simulink model "ExampleAlphaMesh"  (R2024a)
settings: Solver=FixedStepAuto  StartTime=0.0  StopTime=inf  FixedStep=0.02  RelTol=1e-3  EnableMultiTasking=on
undefined symbols (not defined in the file): atmosphericScattering, basicProperties, castShadow, emissionColorMultiplier, meshID, position, quaternion, scale, visible
libraries: PRISMA x14, GenericTarget x1
settings Model: Creator=damerius  LastModifiedBy=Scythe
settings SolverCC: ConcurrentTasks=on  AlgebraicLoopSolver=TrustRegion  PositivePriorityOrder=on
settings DataIOCC: SaveOutput=off  SignalLogging=off  DSMLogging=off  SaveTime=off  ReturnWorkspaceOutputs=off
settings OptimizationCC: DefaultParameterBehavior=Inlined  ReuseModelBlockBuffer=off  ZeroExternalMemoryAtStartup=off  ZeroInternalMemoryAtStartup=off  SimCompilerOptimization=on
settings DebuggingCC: UnconnectedInputMsg=warning  UnconnectedOutputMsg=warning  UnconnectedLineMsg=warning
settings HardwareCC: ProdBitPerLong=64  ProdHWDeviceType=Intel->x86-64 (Linux 64)
settings ModelReferenceCC: EnableRefExpFcnMdlSchedulingChecks=on
settings SFSimCC: SimParseCustomCode=off  SimGenImportedTypeDefs=on  SimTargetLang=C++
settings RTWCC: GenCodeOnly=on  PackageGeneratedCodeAndArtifacts=on  PackageName=PackNGo  RTWVerbose=off  BuildConfiguration=Faster Runs  TargetLang=C++  GPUComputeCapability=3.5  DLArmComputeVersion=19.05
settings CodeAppCC: ForceParamTrailComments=on  MaxIdLength=95  MATLABSourceComments=on  UseSimReservedNames=on
settings GRTTargetCC: TargetLangStandard=C++11 (ISO)  GenerateFullHeader=off  MatFileLogging=off  CodeInterfacePackaging=C++ class

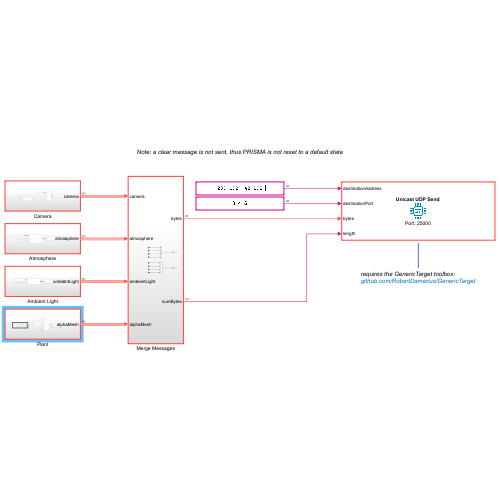
[thumbnail: Simulink's stored preview of the top-level diagram]
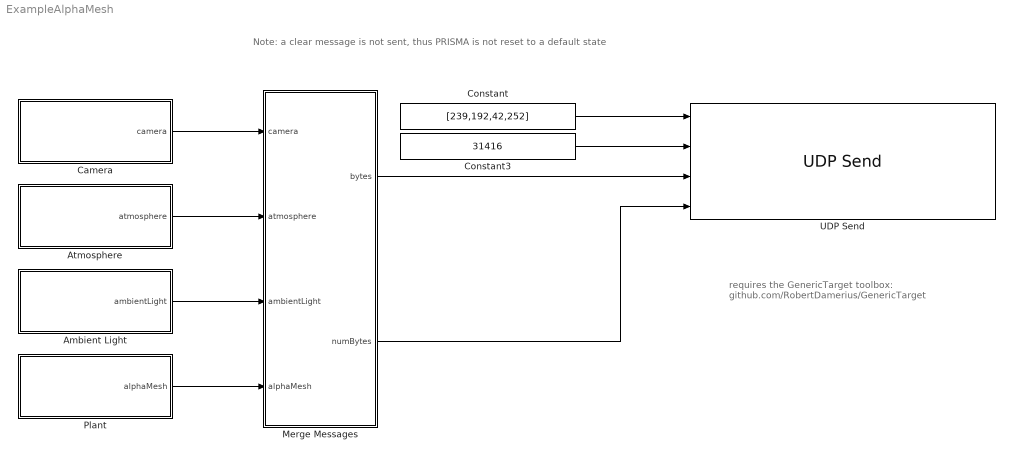
== system ExampleAlphaMesh ==
  note: Note: a clear message is not sent, thus PRISMA is not reset to a default state
  note: requires the GenericTarget toolbox:
      | github.com/RobertDamerius/GenericTarget
  Ambient Light : Subsystem
  Atmosphere : Subsystem
  Camera : Subsystem
  Constant : Constant  Value=[239,192,42,252]  OutDataTypeStr=uint8
  Constant3 : Constant  Value=31416  OutDataTypeStr=uint16
  Merge Messages : Subsystem
  Plant : Subsystem
  UDP Send : GenericTarget/Interface/UDP Send  showDetails=off  interfacePort=25000  interfaceIP=[0,0,0,0]  deviceName=''  prioritySocket=6  allowBroadcast=off  SampleTime=-1
      settings: SourceProductName=Generic Target
  wires:
  Constant3/1 -> UDP Send/2
  Camera/1(camera) -> Merge Messages/1(camera)
  Plant/1(alphaMesh) -> Merge Messages/4(alphaMesh)
  Merge Messages/1(bytes) -> UDP Send/3
  Merge Messages/2(numBytes) -> UDP Send/4
  Ambient Light/1(ambientLight) -> Merge Messages/3(ambientLight)
  Constant/1 -> UDP Send/1
  Atmosphere/1(atmosphere) -> Merge Messages/2(atmosphere)

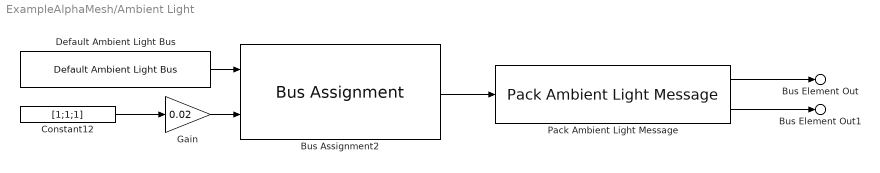
== system ExampleAlphaMesh/Ambient Light ==
  Bus Assignment2 : BusAssignment  AssignedSignals=color
  Constant12 : Constant  Value=[1;1;1]
  Default Ambient Light Bus : PRISMA/Default Ambient Light Bus
      settings: SourceProductName=PRISMA
  Gain : Gain  Gain=0.02
  Pack Ambient Light Message : PRISMA/Pack Ambient Light Message
      settings: SourceProductName=PRISMA
  Bus Element Out : Outport  PortName=ambientLight  Element=bytes
  Bus Element Out1 : Outport  PortName=ambientLight  Element=numBytes
  wires:
  Pack Ambient Light Message/2 -> Bus Element Out1/1
  Pack Ambient Light Message/1 -> Bus Element Out/1
  Gain/1 -> Bus Assignment2/2
  Constant12/1 -> Gain/1
  Default Ambient Light Bus/1 -> Bus Assignment2/1
  Bus Assignment2/1 -> Pack Ambient Light Message/1

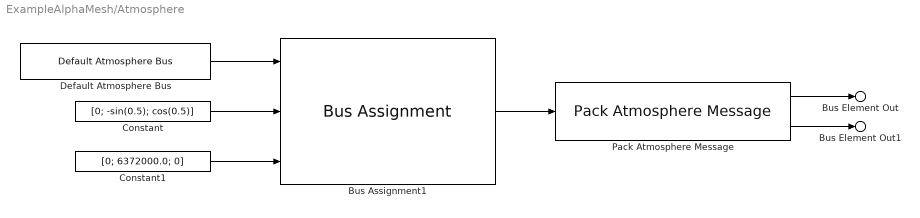
== system ExampleAlphaMesh/Atmosphere ==
  Bus Assignment1 : BusAssignment  AssignedSignals=basicProperties.sunLightDirection,atmosphericScattering.eyePosition
  Constant : Constant  Value=[0; -sin(0.5); cos(0.5)]
  Constant1 : Constant  Value=[0; 6372000.0; 0]
  Default Atmosphere Bus : PRISMA/Default Atmosphere Bus
      settings: SourceProductName=PRISMA
  Pack Atmosphere Message : PRISMA/Pack Atmosphere Message
      settings: SourceProductName=PRISMA
  Bus Element Out : Outport  PortName=atmosphere  Element=bytes
  Bus Element Out1 : Outport  PortName=atmosphere  Element=numBytes
  wires:
  Bus Assignment1/1 -> Pack Atmosphere Message/1
  Default Atmosphere Bus/1 -> Bus Assignment1/1
  Pack Atmosphere Message/1 -> Bus Element Out/1
  Pack Atmosphere Message/2 -> Bus Element Out1/1
  Constant/1 -> Bus Assignment1/2
  Constant1/1 -> Bus Assignment1/3

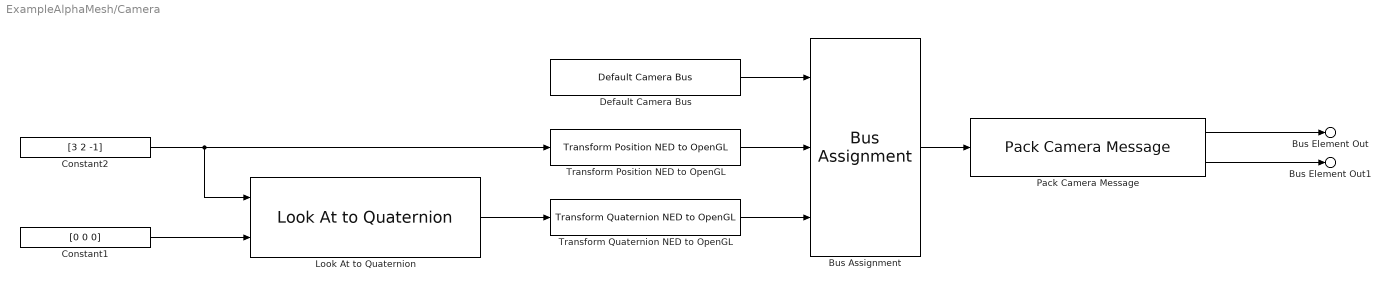
== system ExampleAlphaMesh/Camera ==
  Bus Assignment : BusAssignment  AssignedSignals=position,quaternion
  Constant1 : Constant  Value=[0 0 0]
  Constant2 : Constant  Value=[3 2 -1]
  Default Camera Bus : PRISMA/Default Camera Bus
      settings: SourceProductName=PRISMA
  Look At to Quaternion : PRISMA/Transformation/Look At to Quaternion
      settings: SourceProductName=PRISMA
  Pack Camera Message : PRISMA/Pack Camera Message
      settings: SourceProductName=PRISMA
  Transform Position NED to OpenGL : PRISMA/Transformation/Transform Position NED to OpenGL
      settings: SourceProductName=PRISMA
  Transform Quaternion NED to OpenGL : PRISMA/Transformation/Transform Quaternion NED to OpenGL
      settings: SourceProductName=PRISMA
  Bus Element Out : Outport  PortName=camera  Element=bytes
  Bus Element Out1 : Outport  PortName=camera  Element=numBytes
  wires:
  Default Camera Bus/1 -> Bus Assignment/1
  Bus Assignment/1 -> Pack Camera Message/1
  Transform Position NED to OpenGL/1 -> Bus Assignment/2
  Transform Quaternion NED to OpenGL/1 -> Bus Assignment/3
  Look At to Quaternion/1 -> Transform Quaternion NED to OpenGL/1
  Constant1/1 -> Look At to Quaternion/2
  Pack Camera Message/1 -> Bus Element Out/1
  Pack Camera Message/2 -> Bus Element Out1/1
  Constant2/1 -> Look At to Quaternion/1, Transform Position NED to OpenGL/1

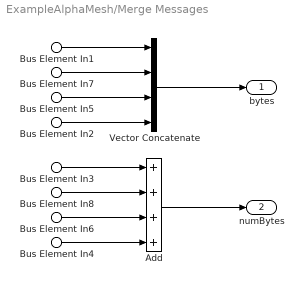
== system ExampleAlphaMesh/Merge Messages ==
  Bus Element In1 : Inport  PortName=camera  Element=bytes
  Bus Element In3 : Inport  PortName=camera  Element=numBytes
  Bus Element In7 : Inport  Port=2  PortName=atmosphere  Element=bytes
  Bus Element In8 : Inport  Port=2  PortName=atmosphere  Element=numBytes
  Bus Element In5 : Inport  Port=3  PortName=ambientLight  Element=bytes
  Bus Element In6 : Inport  Port=3  PortName=ambientLight  Element=numBytes
  Bus Element In2 : Inport  Port=4  PortName=alphaMesh  Element=bytes
  Bus Element In4 : Inport  Port=4  PortName=alphaMesh  Element=numBytes
  Add : Sum  Inputs=++++
  Vector Concatenate : Concatenate  NumInputs=4
  bytes : Outport
  numBytes : Outport  Port=2
  wires:
  Bus Element In1/1 -> Vector Concatenate/1
  Bus Element In2/1 -> Vector Concatenate/4
  Bus Element In3/1 -> Add/1
  Bus Element In4/1 -> Add/4
  Vector Concatenate/1 -> bytes/1
  Add/1 -> numBytes/1
  Bus Element In5/1 -> Vector Concatenate/3
  Bus Element In6/1 -> Add/3
  Bus Element In7/1 -> Vector Concatenate/2
  Bus Element In8/1 -> Add/2

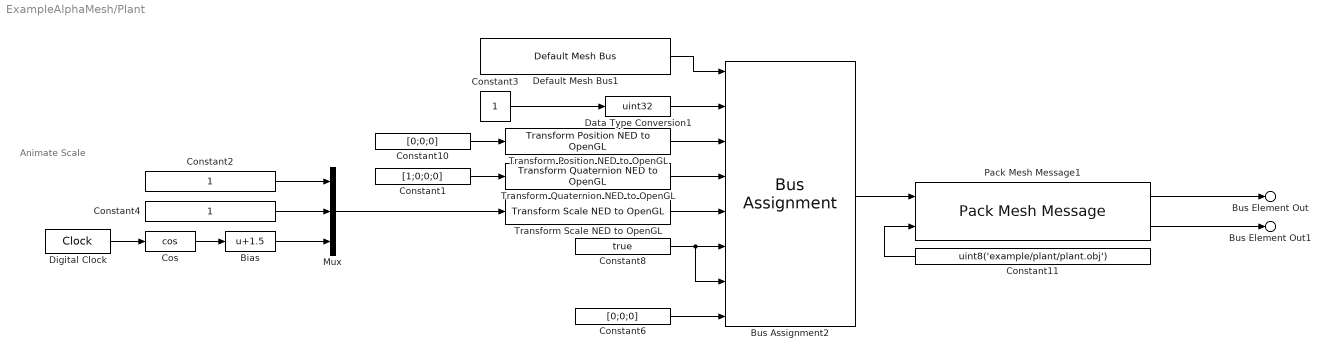
== system ExampleAlphaMesh/Plant ==
  note: Animate Scale
  Bias : Bias  Bias=1.5  SaturateOnIntegerOverflow=off
  Bus Assignment2 : BusAssignment  AssignedSignals=meshID,position,quaternion,scale,visible,castShadow,emissionColorMultiplier
  Constant1 : Constant  Value=[1;0;0;0]
  Constant10 : Constant  Value=[0;0;0]
  Constant11 : Constant  Value=uint8('example/plant/plant.obj')  OutDataTypeStr=uint8
  Constant2 : Constant
  Constant3 : Constant
  Constant4 : Constant
  Constant6 : Constant  Value=[0;0;0]
  Constant8 : Constant  Value=true  OutDataTypeStr=boolean
  Cos : Trigonometry  Operator=cos
  Data Type Conversion1 : DataTypeConversion  OutDataTypeStr=uint32  SaturateOnIntegerOverflow=off  RndMeth=Floor
  Default Mesh Bus1 : PRISMA/Default Mesh Bus
      settings: SourceProductName=PRISMA
  Digital Clock : DigitalClock  SampleTime=0.02
  Mux : Mux  Inputs=3
  Pack Mesh Message1 : PRISMA/Pack Mesh Message
      settings: SourceProductName=PRISMA
  Transform Position NED to OpenGL : PRISMA/Transformation/Transform Position NED to OpenGL
      settings: SourceProductName=PRISMA
  Transform Quaternion NED to OpenGL : PRISMA/Transformation/Transform Quaternion NED to OpenGL
      settings: SourceProductName=PRISMA
  Transform Scale NED to OpenGL : PRISMA/Transformation/Transform Scale NED to OpenGL
      settings: SourceProductName=PRISMA
  Bus Element Out : Outport  PortName=alphaMesh  Element=bytes
  Bus Element Out1 : Outport  PortName=alphaMesh  Element=numBytes
  wires:
  Transform Quaternion NED to OpenGL/1 -> Bus Assignment2/4
  Transform Scale NED to OpenGL/1 -> Bus Assignment2/5
  Constant10/1 -> Transform Position NED to OpenGL/1
  Transform Position NED to OpenGL/1 -> Bus Assignment2/3
  Constant11/1 -> Pack Mesh Message1/2
  Default Mesh Bus1/1 -> Bus Assignment2/1
  Bus Assignment2/1 -> Pack Mesh Message1/1
  Data Type Conversion1/1 -> Bus Assignment2/2
  Constant3/1 -> Data Type Conversion1/1
  Constant6/1 -> Bus Assignment2/8
  Pack Mesh Message1/1 -> Bus Element Out/1
  Pack Mesh Message1/2 -> Bus Element Out1/1
  Constant1/1 -> Transform Quaternion NED to OpenGL/1
  Bias/1 -> Mux/3
  Cos/1 -> Bias/1
  Digital Clock/1 -> Cos/1
  Constant8/1 -> Bus Assignment2/7, Bus Assignment2/6
  Constant2/1 -> Mux/1
  Constant4/1 -> Mux/2
  Mux/1 -> Transform Scale NED to OpenGL/1
